simulink model "Pure_pursuit_by_preview_chord_length"  (R2021a)
settings: configuration reference "AION_IDS_Speedgoat" (kept outside this file)
libraries: simulink x1
settings Model: DataDictionary=Pure_Pursuit_By_Preview_Chord_Length.sldd  Creator=xinrui  LastModifiedBy=Administrator
settings ConfigSetRef: SourceName=AION_IDS_Speedgoat

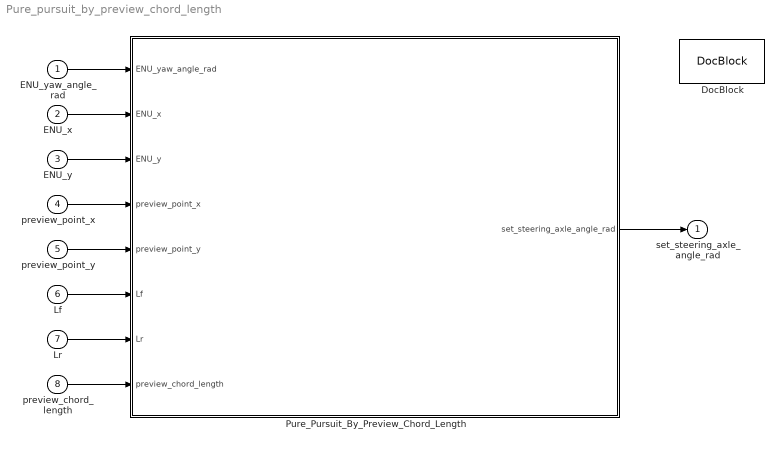
== system Pure_pursuit_by_preview_chord_length ==
  ENU_yaw_angle_rad : Inport  OutDataTypeStr=double  PortDimensions=1
  ENU_x : Inport  Port=2  OutDataTypeStr=double  PortDimensions=1
  ENU_y : Inport  Port=3  OutDataTypeStr=double  PortDimensions=1
  preview_point_x : Inport  Port=4  OutDataTypeStr=double  PortDimensions=1
  preview_point_y : Inport  Port=5  OutDataTypeStr=double  PortDimensions=1
  Lf : Inport  Port=6  OutDataTypeStr=double  PortDimensions=1
  Lr : Inport  Port=7  OutDataTypeStr=double  PortDimensions=1
  preview_chord_length : Inport  Port=8  OutDataTypeStr=double  PortDimensions=1
  DocBlock : simulink/Model-Wide Utilities/DocBlock  DocumentType=HTML  mask(DocBlock){}
      mask Display:
      | plot([.8 0 0 1 1 .8 .8 1],[1 1 0 0 .8 1 .8 .8]);
      | text(.5,.6,'CHANGELOG','horizontalalignment','center');
      | text(.95,.05,get_param(gcb,'DocumentType'),'verticalalignment','bottom','horizontalalignment','right');
  Pure_Pursuit_By_Preview_Chord_Length : MATLAB Function  TreatAsAtomicUnit=on
  set_steering_axle_angle_rad : Outport  OutDataTypeStr=double  PortDimensions=1
  wires:
  ENU_yaw_angle_rad/1 -> Pure_Pursuit_By_Preview_Chord_Length/1(ENU_yaw_angle_rad)
  ENU_x/1 -> Pure_Pursuit_By_Preview_Chord_Length/2(ENU_x)
  ENU_y/1 -> Pure_Pursuit_By_Preview_Chord_Length/3(ENU_y)
  preview_point_x/1 -> Pure_Pursuit_By_Preview_Chord_Length/4(preview_point_x)
  preview_point_y/1 -> Pure_Pursuit_By_Preview_Chord_Length/5(preview_point_y)
  Lf/1 -> Pure_Pursuit_By_Preview_Chord_Length/6(Lf)
  Lr/1 -> Pure_Pursuit_By_Preview_Chord_Length/7(Lr)
  preview_chord_length/1 -> Pure_Pursuit_By_Preview_Chord_Length/8(preview_chord_length)
  Pure_Pursuit_By_Preview_Chord_Length/1(set_steering_axle_angle_rad) -> set_steering_axle_angle_rad/1

== matlab function Pure_pursuit_by_preview_chord_length/Pure_Pursuit_By_Preview_Chord_Length ==
  data: ENU_yaw_angle_rad input double size=1; ENU_x input double size=1; set_steering_axle_angle_rad output double size=1; ENU_y input double size=1; preview_point_x input double size=1; preview_point_y input double size=1; Lf input double size=1; Lr input double size=1; preview_chord_length input double size=1
% 采用预瞄弦长的纯跟踪算法
function set_steering_axle_angle_rad = Pure_pursuit_by_preview_chord_length(...
    ENU_yaw_angle_rad, ENU_x, ENU_y, preview_point_x, preview_point_y, Lf, ...
    Lr, preview_chord_length)
%   1.输入参数：
%       (1)ENU_yaw_angle_rad                    当前车辆在东北天坐标系下的横摆角，rad
%       (2)ENU_x                                当前车辆在东北天坐标系下的x坐标，m
%       (3)ENU_y                                当前车辆在东北天坐标系下的y坐标，m
%       (4)preview_point_x                      预瞄点x坐标，m
%       (5)preview_point_y                      预瞄点y坐标，m
%       (6)Lf                                   前轴距，m
%       (7)Lr                                   后轴距，m
%       (8)preview_chord_length                 预瞄弦长，m
%   2.输出参数：
%       (1)set_steering_axle_angle_rad          目标转向轴转角，rad

%% 将预瞄点坐标从东北天坐标系转换到车辆坐标系下
[x_rotate, y_rotate] = Vehicle_coordinate_transfer_m(ENU_x, ENU_y, ...
    preview_point_x, preview_point_y, ENU_yaw_angle_rad);

%% 求车辆坐标系下预瞄点与原点连线和车辆航向(x轴正方向)的角度偏差alpha，逆时针方向角度为正
alpha = atan(y_rotate / x_rotate);

%% 公式计算求得目标转向轴转角
if 0 < preview_chord_length
    set_steering_axle_angle_rad = atan(2 * (Lf + Lr) * sin(alpha) / preview_chord_length);
else
    set_steering_axle_angle_rad = 0;
end

end
